simulink model "zadz1_sim"  (R2022b)
settings: Solver=VariableStepAuto  StartTime=0.0  StopTime=100  RelTol=1e-3
values from neighbouring files (symbols this model uses):
  c0 = 0.001    [zad1.m]
  q = 0.41625    [zad1.m]
  V = 15.0    (= 15)    [zad1.m]
undefined symbols (not defined in the file or in its folder): sigbuilder_block
settings Model: Creator=DFUNDO  LastModifiedBy=DFUNDO

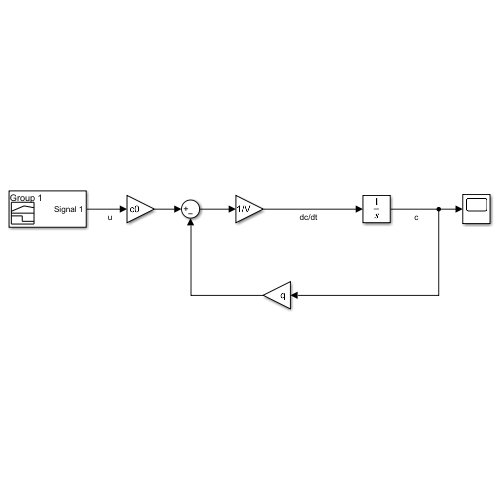
[thumbnail: Simulink's stored preview of the top-level diagram]
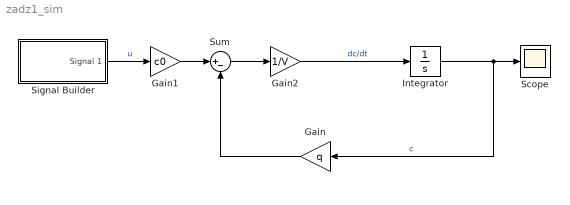
== system zadz1_sim ==
  Gain : Gain  Gain=q
  Gain1 : Gain  Gain=c0
  Gain2 : Gain  Gain=1/V
  Integrator : Integrator
  Scope : Scope
  Signal Builder : Subsystem  Tag=STV Subsys  LoadFcn=sigbuilder_block('load');  StartFcn=sigbuilder_block('start');  StopFcn=sigbuilder_block('stop');  ClipboardFcn=sigbuilder_block('clipboard');  mask(Sigbuilder block){tuvar=[0:10]}
      mask help: Simulink:masks:SigbuilderBlock_MD
      mask init:
      | if ~strcmp(get_param(bdroot(gcbh),'SimulationStatus'),'stopped') tuvar = sigbuilder_block('maskInit'); end
      settings: CopyFcn=sigbuilder_block('copy');  DeleteFcn=sigbuilder_block('delete');  ModelCloseFcn=sigbuilder_block('modelClose');  PreSaveFcn=sigbuilder_block('preSave');  PauseFcn=sigbuilder_block('pause');  ContinueFcn=sigbuilder_block('continue');  NameChangeFcn=sigbuilder_block('namechange');  OpenFcn=sigbuilder_block('open',[232 199.2 756 400 ]);  CloseFcn=sigbuilder_block('close');
      mask Display: plot(0, 0, 100, 100,[2, 2, 32, 32, 2], [68, 8, 8, 68, 68],[32, 2], [38, 38], [32, 19, 2],[53, 60, 44], [32, 17, 17, 2],[16, 16, 31, 31]);txt = getActiveGroup(gcbh);text(2, 100, txt,'verticalAlignment', 'top');
  Sum : Sum  Inputs=|+-
  wires:
  Integrator/1 -> Scope/1, Gain/1  "c"
  Gain2/1 -> Integrator/1  "dc/dt"
  Gain/1 -> Sum/2
  Gain1/1 -> Sum/1
  Signal Builder/1(Signal 1) -> Gain1/1  "u"
  Sum/1 -> Gain2/1

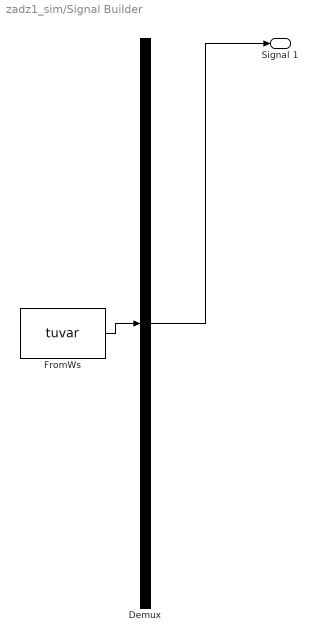
== system zadz1_sim/Signal Builder ==
  Demux : Demux  Tag=STV Demux  Outputs=1
      settings: DisplayOption=none
  FromWs : FromWorkspace  Tag=STV FromWs  VariableName=tuvar
      SigBuilderData=|
      | common.afterFinalStr = 'Extrapolate'
      | common.sampleTime = 0
      | dataSet.timeRange = [0 100]
      | dataSet.name = 'Group 1'
      | sbobj.Groups.Name = 'Group 1'
      | sbobj.Groups.Signals.Name = 'Signal 1'
      | sbobj.Groups.Signals.XData = [0 1.05 1.05 2 2 49 49 50 50 100]
      | sbobj.Groups.Signals.YData = [0.005 0.005 1.005 1.005 0 -0.005 0.995 0.995 0 0]
      | sbobj.Groups.TimeRange = [0 100]
  Signal 1 : Outport  Tag=STV Outport
  wires:
  Demux/1 -> Signal 1/1
  FromWs/1 -> Demux/1
